simulink model "comb_c_noise"  (Simulink 5.0)
settings: Solver=ode23s  StartTime=t0  StopTime=tf  RelTol=1e-8  AbsTol=1.0e-8
values from neighbouring files (symbols this model uses):
  st = 1    [ant-old.m]    (also in ibm_pp.m; motor_pd.m; unstb.m)
  Ts = 0.01; [B,A,k] = myc2d(G,Ts)    [ant-old.m]    (also in ibm_pp.m = 1; motor_pd.m = 0.25; [B,A,k] = myc2d(G,Ts); unstb.m = 1)
undefined symbols (not defined in the file or in its folder): den, num, R, S, tau, TM
settings Model: Creator=kannanm  LastModifiedBy=kannan  ExtModeAutoUpdateStatusClock=off

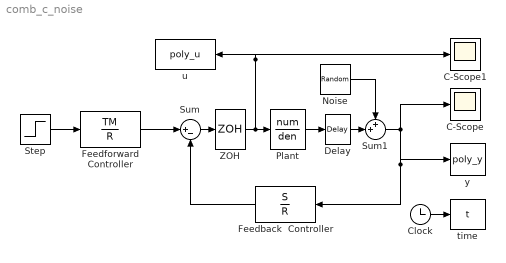
== system comb_c_noise ==
  C-Scope : Scope
      settings: YMin=-5e+13  YMax=4e+14
  C-Scope1 : Scope
      settings: YMin=-3e+14  YMax=3e+14
  Clock : Clock
      settings: Decimation=10
  Delay : TransportDelay  DelayTime=tau
  Feedback  Controller : DiscreteFilter  Orientation=left  Numerator=S  Denominator=R  SampleTime=Ts
  Feedforward Controller : DiscreteFilter  Numerator=TM  Denominator=R  SampleTime=Ts
  Noise : RandomNumber  SampleTime=Ts
  Plant : TransferFcn  Numerator=num  Denominator=den
  Step : Step  Time=0  After=st  SampleTime=Ts
  Sum : Sum  Inputs=|+-  SaturateOnIntegerOverflow=on
  Sum1 : Sum  Inputs=++|  SaturateOnIntegerOverflow=on
  ZOH : ZeroOrderHold  SampleTime=Ts
  time : ToWorkspace  VariableName=t  SampleTime=Ts  SaveFormat=Array
  u : ToWorkspace  VariableName=poly_u  SampleTime=Ts  SaveFormat=Array
  y : ToWorkspace  VariableName=poly_y  SampleTime=Ts  SaveFormat=Array
  wires:
  Step/1 -> Feedforward Controller/1
  Feedforward Controller/1 -> Sum/1
  Sum/1 -> ZOH/1
  Feedback  Controller/1 -> Sum/2
  ZOH/1 -> Plant/1, u/1, C-Scope1/1
  Clock/1 -> time/1
  Plant/1 -> Delay/1
  Delay/1 -> Sum1/2
  Noise/1 -> Sum1/1
  Sum1/1 -> C-Scope/1, Feedback  Controller/1, y/1
